simulink model "simulink "  (R2022b)
settings: Solver=VariableStepAuto  StartTime=0.0  StopTime=400  RelTol=1e-3
values from neighbouring files (symbols this model uses):
  Kp = 7.21    [simulink_data .m]
  Kp1 = 1.9125    [simulink_data .m]
  Ti = 1.66    [simulink_data .m]
  Ti1 = 9.96    [simulink_data .m]
undefined symbols (not defined in the file or in its folder): L1, M1
settings Model: Creator=parince  LastModifiedBy=parince

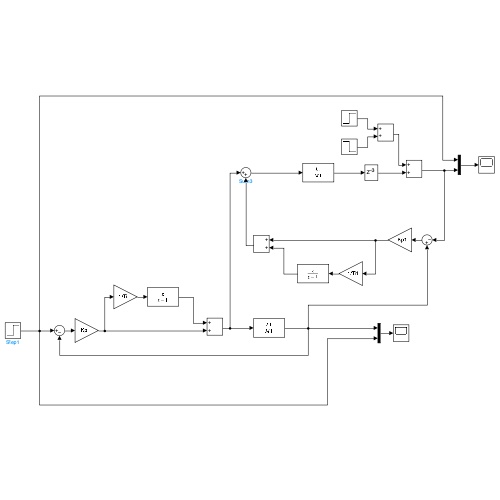
[thumbnail: Simulink's stored preview of the top-level diagram]
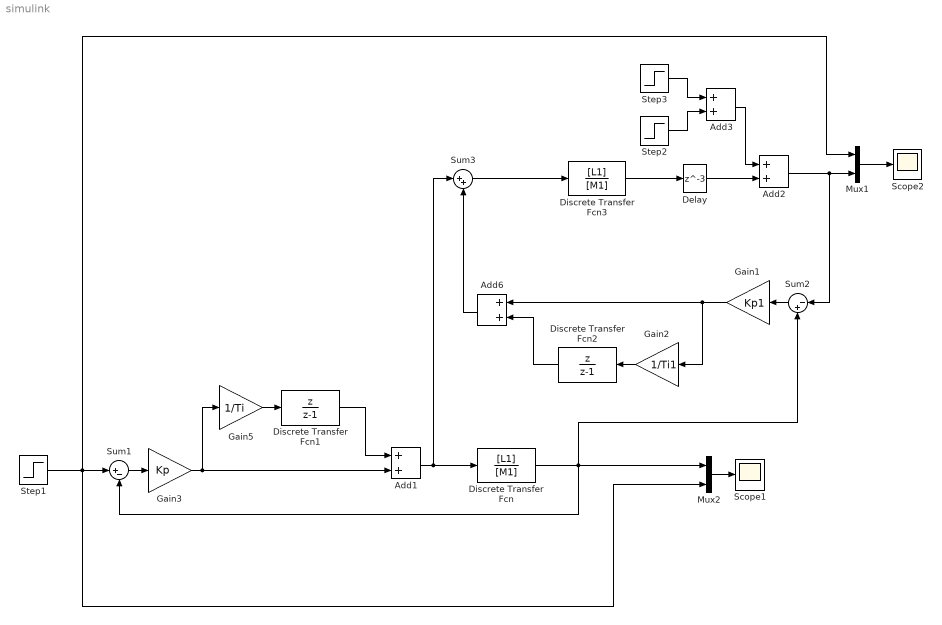
== system simulink  ==
  Add{1..3,6} (4 alike) : Sum
  Delay : Delay  DelayLength=3  InitialCondition=0
  Discrete Transfer Fcn : DiscreteTransferFcn  Numerator=[L1]  Denominator=[M1]  SampleTime=1
  Discrete Transfer Fcn1 : DiscreteTransferFcn  Numerator=[1 0]  Denominator=[1 -1]  SampleTime=1
  Discrete Transfer Fcn2 : DiscreteTransferFcn  Numerator=[1 0]  Denominator=[1 -1]  SampleTime=1
  Discrete Transfer Fcn3 : DiscreteTransferFcn  Numerator=[L1]  Denominator=[M1]  SampleTime=1
  Gain1 : Gain  Gain=Kp1
  Gain2 : Gain  Gain=1/Ti1
  Gain3 : Gain  Gain=Kp
  Gain5 : Gain  Gain=1/Ti
  Mux1 : Mux  Inputs=2
  Mux2 : Mux  Inputs=2
  Scope1 : Scope
  Scope2 : Scope
  Step1 : Step  SampleTime=0
  Step2 : Step  Time=300  After=-0.1  SampleTime=0
  Step3 : Step  Time=200  After=0.1  SampleTime=0
  Sum1 : Sum  Inputs=|+-
  Sum2 : Sum  Inputs=|-+
  Sum3 : Sum  Inputs=|++
  wires:
  Step1/1 -> Mux1/1, Mux2/2, Sum1/1
  Gain5/1 -> Discrete Transfer Fcn1/1
  Sum1/1 -> Gain3/1
  Add1/1 -> Sum3/1, Discrete Transfer Fcn/1
  Gain3/1 -> Gain5/1, Add1/2
  Mux2/1 -> Scope1/1
  Discrete Transfer Fcn/1 -> Sum2/2, Mux2/1, Sum1/2
  Discrete Transfer Fcn1/1 -> Add1/1
  Add2/1 -> Sum2/1, Mux1/2
  Gain2/1 -> Discrete Transfer Fcn2/1
  Discrete Transfer Fcn2/1 -> Add6/2
  Gain1/1 -> Gain2/1, Add6/1
  Add6/1 -> Sum3/2
  Sum3/1 -> Discrete Transfer Fcn3/1
  Sum2/1 -> Gain1/1
  Discrete Transfer Fcn3/1 -> Delay/1
  Mux1/1 -> Scope2/1
  Delay/1 -> Add2/2
  Add3/1 -> Add2/1
  Step3/1 -> Add3/1
  Step2/1 -> Add3/2
